simulink model "emergency_generator"  (R2014a)
settings: Solver=ode23tb  SolverMode=SingleTasking  StartTime=0.0  StopTime=10  RelTol=1e-4
undefined symbols (not defined in the file or in its folder): D1, Delta
libraries: powerlib x11, sps_avr x1
Description:
  | Copyright 2008-2014 The MathWorks, Inc.
settings Model: FPTRunName=Active  ExtModeTrigMode=oneshot  ExtModeArmWhenConnect=off  ExtModeAutoUpdateStatusClock=off  Creator=MathWorks  LastModifiedBy=cosorio
settings SolverCC: ZeroCrossAlgorithm=Adaptive
settings DataIOCC: LimitDataPoints=off  SaveOutput=off  SaveTime=off  SignalLoggingName=sigsOut  OutputTimes=[0:1/20:10]
settings OptimizationCC: BlockReduction=off  BooleanDataType=off  ExpressionDepthLimit=2147483647  InitFltsAndDblsToZero=on  EfficientMapNaN2IntZero=off
settings DebuggingCC: UnderspecifiedInitializationDetection=Classic  CheckExecutionContextPreStartOutputMsg=on  CheckExecutionContextRuntimeOutputMsg=on  SignalResolutionControl=TryResolveAllWithWarning  IgnoredZcDiagnostic=none  SolverPrmCheckMsg=none  MultiTaskDSMMsg=warning  MultiTaskCondExecSysMsg=none  SigSpecEnsureSampleTimeMsg=none  FcnCallInpInsideContextMsg=UseLocalSettings  UnconnectedInputMsg=none  UnconnectedOutputMsg=none  UnconnectedLineMsg=none  StateNameClashWarn=warning
settings HardwareCC: ProdHWDeviceType=Specified  TargetUnknown=on
settings RTWCC: IncludeERTFirstTime=on
settings CodeAppCC: IgnoreCustomStorageClasses=off
settings GRTTargetCC: TargetFcnLib=ansi_tfl_tmw.mat  CombineOutputUpdateFcns=off  GRTInterface=on

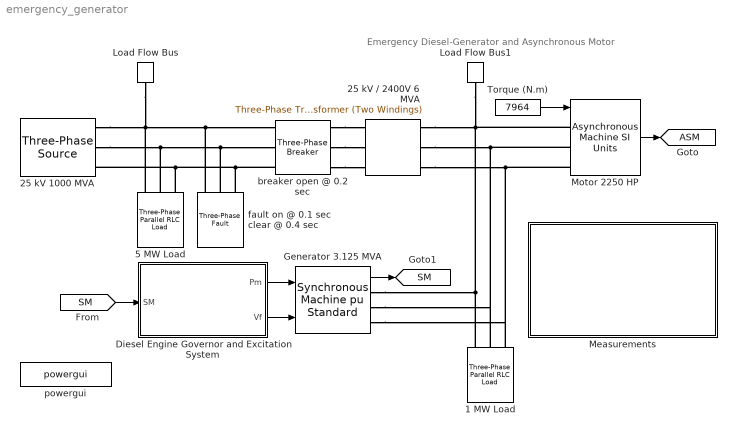
== system emergency_generator ==
  note: Emergency Diesel-Generator and Asynchronous Motor
  1 MW Load : powerlib/Elements/Three-Phase Parallel RLC Load  LConnTagsString=A|B|C  Configuration=Y (grounded)  NominalVoltage=2400  NominalFrequency=60  ActivePower=1e+006  InductivePower=0  CapacitivePower=0  Measurements=None  LoadType=constant Z
  25 kV 1000 MVA : powerlib/Electrical Sources/Three-Phase Source  Voltage=25000  PhaseAngle=2.1395e-05  Frequency=60  InternalConnection=Yg  SpecifyImpedance=on  Resistance=25^2/1000/10  Inductance=25^2/1000/377  ShortCircuitLevel=1000e6  BaseVoltage=25e3  XRratio=10  BusType=swing  Pref=0  Qref=0  Qmin=-Inf  Qmax=Inf
  25 kV / 2400V 6 MVA : powerlib/Elements/Three-Phase Transformer (Two Windings)  Winding1Connection=Yg  UNITS=pu  NominalPower=[ 6e6 , 60 ]  Winding1=[ 25e3 , 0.0015 , 0.03]  Winding2Connection=Delta (D1)  Winding2=[ 2.4e3 , 0.0015 , 0.03 ]  SetSaturation=off  Rm=200  Lm=200  Saturation="[ 0,0  ;  0.005,1.2  ;  1.0,1.4 ]"  Hysteresis=off  DataFile='hysteresis'  SetInitialFlux=off  InitialFluxes=[ 0.8 , -0.8 , 0.7 ]  Measurements=None  MoreParameters=off  BreakLoop=off  DataType=off  TransfoNumber=0
  5 MW Load : powerlib/Elements/Three-Phase Parallel RLC Load  LConnTagsString=A|B|C  Configuration=Y (grounded)  NominalVoltage=25e3  NominalFrequency=60  ActivePower=5e+006  InductivePower=0  CapacitivePower=0  Measurements=None  LoadType=constant Z
  Diesel Engine Governor and Excitation System : Subsystem
  Generator 3.125 MVA : powerlib/Machines/Synchronous Machine pu Standard  PresetModel=No  MechanicalLoad=Mechanical power Pm  ShowDetailedParameters=on  RotorType=Salient-pole  Units=per unit standard parameters  MeasurementBus=off  NominalParameters="[ 3.125e6  2400  60]"  Reactances1=[ 31 32 33 34 35 36 37 ]  Reactances2=[ 1.56, 0.296, 0.177, 1.06, 0.177, 0.052 ]  dAxisTimeConstants=Short-circuit  qAxisTimeConstants=Open-circuit  TimeConstants1=[]  TimeConstants2=[]  TimeConstants3=[]  TimeConstants4=[]  TimeConstants5=[ 3.7, 0.05, 0.05 ]  TimeConstants6=[ 8.0, 0.03, 0.3371, 0.0295 ]  TimeConstants7=[0.024 0.006 0.006]  TimeConstants8=[]  StatorResistance=0.0036  Mechanical="[ 1.07  0 2]"  PolePairs=2  InitialConditions=[0 0 0 0 0 0 0 0 1]  SetSaturation=off  Saturation=[0.211 0.418 1.0 1.25 1.72 3.35 ;0.25 0.50 1.0 1.1 1.2 1.4]  LoadFlowParameters=[1 0 0 0]  TsPowergui=0  TsBlock=-1  IterativeModel=Forward Euler  BusType=PV  Pref=0  Qref=0  Qmin=-Inf  Qmax=Inf  PLF=0  QLF=0
      settings: AttributesFormatString=\n\n
  Load Flow Bus : powerlib/Measurements/Load Flow Bus  LConnTagsString=a  ID=B1  Vbase=25e3  Vref=1  Vangle=0  VLF=1  angleLF=0
      settings: AttributesFormatString=%<ID>\n%<Vbase>V\n%<VLF>pu\n%<angleLF>deg.
  Load Flow Bus1 : powerlib/Measurements/Load Flow Bus  LConnTagsString=a  ID=B2  Vbase=2400  Vref=1  Vangle=0  VLF=1  angleLF=0
      settings: AttributesFormatString=%<ID>\n%<Vbase>V\n%<VLF>pu\n%<angleLF>deg.
  Measurements : Subsystem
  Motor 2250 HP : powerlib/Machines/Asynchronous Machine SI Units  PresetModel=No  MechanicalLoad=Torque Tm  ShowDetailedParameters=on  RotorType=Squirrel-cage  ReferenceFrame=Rotor  Units=SI  MeasurementBus=off  NominalParameters=[2250*746, 2400, 60 ]  Stator=[ 0.029 0.226/377]  Rotor=[ 0.022 0.226/377]  Cage1=[ 0.022 0.226/377]  Cage2=[ 0.022 0.226/377]  Lm=13.04/377  Mechanical=[ 63.87 0 2]  PolePairs=2  InitialConditions=[0 0 0 0 0 0 0 0]  SimulateSaturation=off  Saturation=[14.03593122, 27.81365428, 53.79336849, 72.68890987, 97.98006896, 148.6815601, 215.7428561, 302.9841135, 428.7778367 ; 230, 322, 414, 460, 506, 552, 598, 644, 690]  LoadFlowParameters=1492000  TsPowergui=0  TsBlock=-1  IterativeModel=Forward Euler  Pmec=1.492e6
  Torque (N.m) : Constant  Value=7964
  breaker open @ 0.2 sec : powerlib/Elements/Three-Phase Breaker  InitialState=closed  SwitchA=on  SwitchB=on  SwitchC=on  SwitchTimes=[0.2]  External=off  BreakerResistance=0.01  SnubberResistance=1e5  SnubberCapacitance=inf  Measurements=None
      settings: AttributesFormatString=\n
  fault on @ 0.1 sec clear @ 0.4 sec : powerlib/Elements/Three-Phase Fault  InitialStates=0  FaultA=on  FaultB=on  FaultC=on  GroundFault=on  SwitchTimes=[0.1 0.4]  External=off  SwitchStatus=NaN  FaultResistance=0.01  GroundResistance=0.001  SnubberResistance=inf  SnubberCapacitance=inf  Measurements=None
  powergui : powerlib/powergui  Priority=2  SimulationMode=Continuous  SolverType=Tustin  SampleTime=50e-6  frequency=60  SPID=off  DisableSnubberDevices=off  DisableRonSwitches=off  DisableVfSwitches=off  SwTol=0  Interpol=off  DisplayEquations=off  Ts=0  methode=off  frequencyindice=60  Pbase=1e6  ErrMax=0.0001  Iterations=50  UnitsV=kV  UnitsW=MW  FunctionMessages=off  echomessages=off  HookPort=off  EnableUseOfTLC=off  x0status=blocks  RestoreLinks=warning  ResistiveCurrentMeasurement=off  Frange=logspace(0,3,50)  Ylog=off  Xlog=off  ShowGrid=off  save=off  variable=ZData  structure=0  ZoomFFT=on  StartTime=0.0  cycles=2  DisplayStyle=off  fundamental=60  FreqAxis=off  MaxFrequency=1000  frequencyindicesteady=1  RmsSteady=1  display=off
  tag scope: ASM=global, SM=global
  wires:
  Torque (N.m)/1 -> Motor 2250 HP/1
  Motor 2250 HP/1 -> [ASM]
  Generator 3.125 MVA/1 -> [SM]
  Diesel Engine Governor and Excitation System/1(Pm) -> Generator 3.125 MVA/1
  Diesel Engine Governor and Excitation System/2(Vf) -> Generator 3.125 MVA/2
  [SM] -> Diesel Engine Governor and Excitation System/1(SM)
  connections:
  Motor 2250 HP/LConn2 -- 25 kV / 2400V 6 MVA/RConn2 -- Generator 3.125 MVA/RConn2 -- 1 MW Load/LConn2
  Motor 2250 HP/LConn3 -- 25 kV / 2400V 6 MVA/RConn3 -- Generator 3.125 MVA/RConn3 -- 1 MW Load/LConn3
  breaker open @ 0.2 sec/RConn1 -- 25 kV / 2400V 6 MVA/LConn1
  breaker open @ 0.2 sec/RConn2 -- 25 kV / 2400V 6 MVA/LConn2
  breaker open @ 0.2 sec/RConn3 -- 25 kV / 2400V 6 MVA/LConn3
  25 kV 1000 MVA/RConn1 -- Load Flow Bus/LConn1 -- 5 MW Load/LConn1 -- fault on @ 0.1 sec clear @ 0.4 sec/LConn1 -- breaker open @ 0.2 sec/LConn1
  breaker open @ 0.2 sec/LConn3 -- 25 kV 1000 MVA/RConn3 -- 5 MW Load/LConn3 -- fault on @ 0.1 sec clear @ 0.4 sec/LConn3
  25 kV 1000 MVA/RConn2 -- 5 MW Load/LConn2 -- breaker open @ 0.2 sec/LConn2 -- fault on @ 0.1 sec clear @ 0.4 sec/LConn2
  Generator 3.125 MVA/RConn1 -- 1 MW Load/LConn1 -- Load Flow Bus1/LConn1 -- 25 kV / 2400V 6 MVA/RConn1 -- Motor 2250 HP/LConn1

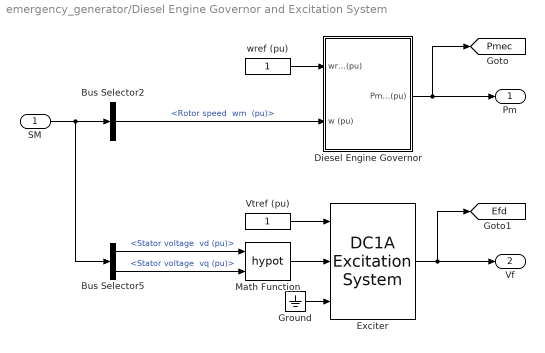
== system emergency_generator/Diesel Engine Governor and Excitation System ==
  SM : Inport
  Bus Selector2 : BusSelector  OutputSignals="Mechanical.Rotor speed  wm  (pu)"
  Bus Selector5 : BusSelector  OutputSignals="dq0 components.Stator voltage  vd (pu),dq0 components.Stator voltage  vq (pu)"
  Diesel Engine Governor : Subsystem  mask(Diesel Engine & Governor){K=40, Tr=[0.01 0.02 0.2], Ta=[0.25 0.009 0.0384], Tlim=[0 1.1], Td=0.024, Pm0=0}
      mask prompts: K "Regulator gain K:"; Tr "Regulator time constants [T1 T2 T3 ] (s) :"; Ta "Actuator time constants [T4 T5 T6] (s) :"; Tlim "Torque limits [Tmin Tmax] (pu) :"; Td "Engine time delay Td (s) :"; Pm0 "Initial value of mechanical power  Pm0 (pu) :"
      mask help:
      | This block implements a diesel engine and governor system:
      | 1st and 2nd inputs: Desired and actual speed (pu)
      | Output: Diesel engine mechanical power.Motor inertia should be combined with generator.
      | Controller transfer function:
      |      Hc=K.(1+T3.s)/(1+T1.s+T1.T2.s^2)
      | Actuator transfer function :
      |      Ha= (1+T4.s) / [ (s (1+T5.s)(1+T6.s) ]
      | Motor :
      |      Time delay Td
      |
      | (See reference in Tutorial Session 5)
  Exciter : sps_avr/DC1A Excitation System  Tr=20e-3  KaTa=[46 0.06]  VRminmax=[-0.9 1.0]  KfTf=[0.05 1.5]  TbTc=[0 0]  KeTe=[0.05 0.46]  Efd12=[3.1 2.3]  SeEfd12=[0.33 0.10]  v0=[1 0]  TsBlock=-2
  Ground : Ground
  Math Function : Math  Operator=hypot  SaturateOnIntegerOverflow=on
  "Vtref (pu) " : Constant
  wref (pu) : Constant
  Pm : Outport
  Vf : Outport  Port=2
  tag scope: Efd=global, Pmec=global
  wires:
  Bus Selector5/1 -> Math Function/1  "<Stator voltage  vd (pu)>"
  Math Function/1 -> Exciter/2
  SM/1 -> Bus Selector5/1, Bus Selector2/1
  Bus Selector5/2 -> Math Function/2  "<Stator voltage  vq (pu)>"
  Diesel Engine Governor/1(Pmec (pu)) -> [Pmec], Pm/1
  Bus Selector2/1 -> Diesel Engine Governor/2(w (pu))  "<Rotor speed  wm  (pu)>"
  "Vtref (pu) "/1 -> Exciter/1
  wref (pu)/1 -> Diesel Engine Governor/1(wref (pu))
  Exciter/1 -> [Efd], Vf/1
  Ground/1 -> Exciter/3

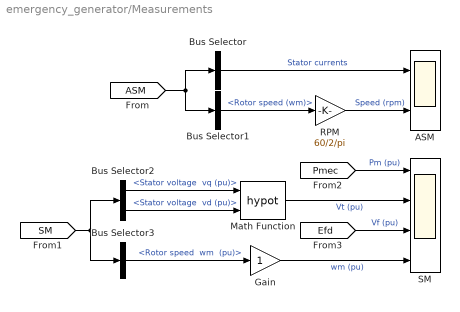
== system emergency_generator/Measurements ==
  ASM : Scope  NumInputPorts=2
      settings: YMin=-2000~1600  YMax=2000~1800  SaveName=ASMData
  Bus Selector : BusSelector  OutputSignals=Stator measurements.Stator current is_a (A),Stator measurements.Stator current is_b (A),Stator measurements.Stator current is_c (A)  OutputAsBus=on
  Bus Selector1 : BusSelector  OutputSignals=Mechanical.Rotor speed (wm)
  Bus Selector2 : BusSelector  OutputSignals="dq0 components.Stator voltage  vq (pu),dq0 components.Stator voltage  vd (pu)"
  Bus Selector3 : BusSelector  OutputSignals="Mechanical.Rotor speed  wm  (pu)"
  Gain : Gain
  Math Function : Math  Operator=hypot  SaturateOnIntegerOverflow=on
  RPM : Gain  Gain=60/2/pi  SaturateOnIntegerOverflow=on  OutDataTypeStr=Inherit: Same as input  ParamDataTypeStr=Inherit: Same as input
  SM : Scope  NumInputPorts=4
      settings: YMin=0~0~0~0.96  YMax=1~1.5~4~1.04  SaveName=SMData  DataFormat=Structure
  wires:
  Bus Selector/1 -> ASM/1  "Stator currents"
  Bus Selector1/1 -> RPM/1  "<Rotor speed (wm)>"
  RPM/1 -> ASM/2  "Speed (rpm)"
  [ASM] -> Bus Selector/1, Bus Selector1/1
  [SM] -> Bus Selector3/1, Bus Selector2/1
  Bus Selector2/1 -> Math Function/1  "<Stator voltage  vq (pu)>"
  Bus Selector2/2 -> Math Function/2  "<Stator voltage  vd (pu)>"
  Bus Selector3/1 -> Gain/1  "<Rotor speed  wm  (pu)>"
  [Pmec] -> SM/1  "Pm (pu)"
  Gain/1 -> SM/4  "wm (pu)"
  [Efd] -> SM/3  "Vf (pu)"
  Math Function/1 -> SM/2  "Vt (pu)"

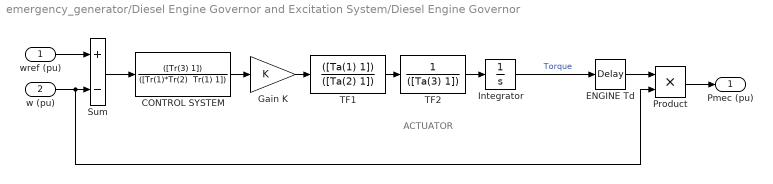
== system emergency_generator/Diesel Engine Governor and Excitation System/Diesel Engine Governor ==
  note: ACTUATOR
  wref (pu) : Inport
  w (pu) : Inport  Port=2
  CONTROL SYSTEM : TransferFcn  Numerator=([Tr(3) 1])  Denominator="([Tr(1)*Tr(2)  Tr(1) 1])"
  ENGINE Td : TransportDelay  DelayTime=Td  InitialOutput=Pm0
  Gain K : Gain  Gain=K  SaturateOnIntegerOverflow=on  OutDataTypeStr=Inherit: Same as input  ParamDataTypeStr=Inherit: Same as input
  Integrator : Integrator  InitialCondition=Pm0  LimitOutput=on  UpperSaturationLimit=Tlim(2)  LowerSaturationLimit=Tlim(1)
  Product : Product  SaturateOnIntegerOverflow=on  InputSameDT=on  OutDataTypeStr=Inherit: Same as first input
  Sum : Sum  Inputs=+-  SaturateOnIntegerOverflow=on  InputSameDT=on  OutDataTypeStr=Inherit: Same as first input
  TF1 : TransferFcn  Numerator=([Ta(1) 1])  Denominator=([Ta(2) 1])
  TF2 : TransferFcn  Numerator=1  Denominator=([Ta(3) 1])
  Pmec (pu) : Outport  InitialOutput=0
  wires:
  Integrator/1 -> ENGINE Td/1  "Torque"
  TF2/1 -> Integrator/1
  Product/1 -> Pmec (pu)/1
  wref (pu)/1 -> Sum/1
  ENGINE Td/1 -> Product/1
  w (pu)/1 -> Sum/2, Product/2
  TF1/1 -> TF2/1
  CONTROL SYSTEM/1 -> Gain K/1
  Sum/1 -> CONTROL SYSTEM/1
  Gain K/1 -> TF1/1
